simulink model "Vending_machine"  (R2020b)
settings: Solver=VariableStepAuto  StartTime=0.0  StopTime=300.0  RelTol=1e-3
settings Model: Creator=JAGRUTI SHINDE  LastModifiedBy=JAGRUTI SHINDE

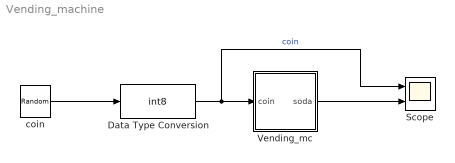
== system Vending_machine ==
  Data Type Conversion : DataTypeConversion  OutDataTypeStr=int8  RndMeth=Nearest
  Scope : Scope  NumInputPorts=2
  Vending_mc : Stateflow chart  TreatAsAtomicUnit=on
  coin : UniformRandomNumber  Minimum=0  Maximum=2  Seed=337  SampleTime=10
  wires:
  Vending_mc/1(soda) -> Scope/2
  coin/1 -> Data Type Conversion/1
  Data Type Conversion/1 -> Scope/1, Vending_mc/1(coin)  "coin"

== stateflow chart Vending_machine/Vending_mc ==
  state Active_state
  state Nickel_state
  state Dime_state
  (default) -> Active_state
  Active_state -> Nickel_state [order 1] : [coin==1]{soda=0}
  Dime_state -> Active_state [order 1] : [coin==1]{soda=1}
  Active_state -> Dime_state [order 2] : [coin==2]{soda=0}
  Nickel_state -> Active_state [order 2] : [coin==2]{soda=1}
  Dime_state -> Nickel_state [order 2] : [coin==2]{soda=1}
  Nickel_state -> Dime_state [order 1] : [coin==1]{soda=0}
  data: coin input; soda output
